simulink model "Mixture"  (Simulink 6.3)
settings: Solver=ode23s  StartTime=0  StopTime=800  MaxStep=0.1  RelTol=1e-3
undefined symbols (not defined in the file or in its folder): sigbuilder_block
Description:
  | This is a model of depression in synapses
settings Model: Creator=chchlee  LastModifiedBy=Owner  ExtModeAutoUpdateStatusClock=off
settings DataIOCC: SignalLoggingName=sigsOut
settings OptimizationCC: InlineInvariantSignals=on
settings DebuggingCC: SolverPrmCheckMsg=none
settings HardwareCC: TargetUnknown=on
settings GRTTargetCC: ModelReferenceCompliant=off  MatFileLogging=off

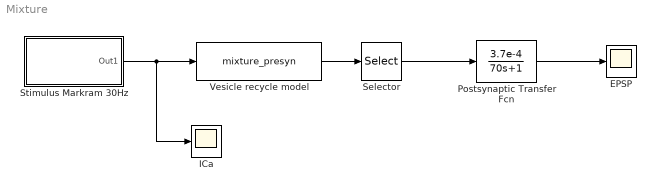
== system Mixture ==
  EPSP : Scope
      settings: TimeRange=600  YMin=-90  YMax=-76  SaveName=sim_mixture  DataFormat=Array
  ICa : Scope
      settings: YMin=-67.5  YMax=-63  SaveName=ScopeData3
  Postsynaptic Transfer Fcn : TransferFcn  Numerator=[3.7e-4]  Denominator=[70 1]
  Selector : Selector  Elements=[4]  InputPortWidth=4
  Stimulus Markram 30Hz : Subsystem
  Vesicle recycle model : S-Function  FunctionName=mixture_presyn
  wires:
  Selector/1 -> Postsynaptic Transfer Fcn/1
  Stimulus Markram 30Hz/1(Out1) -> ICa/1, Vesicle recycle model/1
  Vesicle recycle model/1 -> Selector/1
  Postsynaptic Transfer Fcn/1 -> EPSP/1

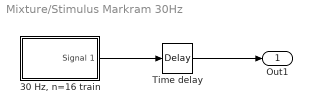
== system Mixture/Stimulus Markram 30Hz ==
  "30 Hz, n=16 train" : Subsystem  Tag=STV Subsys  LoadFcn=sigbuilder_block('load');  StartFcn=sigbuilder_block('start');  StopFcn=sigbuilder_block('stop');  ClipboardFcn=sigbuilder_block('clipboard');  mask(Sigbuilder block){}
      mask help: Sigbuilder GUI
      mask init:
      | if ~strcmp(get_param(bdroot(gcbh),'SimulationStatus'),'stopped') tuvar = sigbuilder_block('maskInit'); end
      settings: CopyFcn=sigbuilder_block('copy');  DeleteFcn=sigbuilder_block('delete');  ModelCloseFcn=sigbuilder_block('modelClose');  PreSaveFcn=sigbuilder_block('preSave');  NameChangeFcn=sigbuilder_block('namechange');  OpenFcn=sigbuilder_block('open',[-3 25.5 768 498 ]);  CloseFcn=sigbuilder_block('close');
      mask Display: plot(0,0,100,100,[10,10,40,40,10],[80,20,20,80,80],[40,10],[50,50], [40,27,10],[65,72,56],[40,25,25,10],[28,28,43,43]);
  Time delay : TransportDelay  DelayTime=60  BufferSize=2000
  Out1 : Outport
  wires:
  "30 Hz, n=16 train"/1(Signal 1) -> Time delay/1
  Time delay/1 -> Out1/1

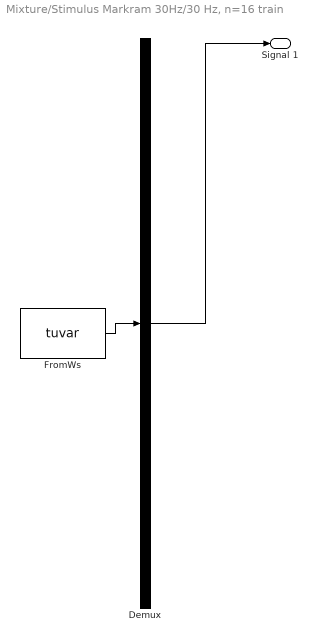
== system Mixture/Stimulus Markram 30Hz/30 Hz, n=16 train ==
  Demux : Demux  Tag=STV Demux  Outputs=1
  FromWs : FromWorkspace  Tag=STV FromWs  VariableName=tuvar  SampleTime=0  SigBuilderData=DataTag0  VnvData=DataTag1
      SigBuilderData=|
      | channels.label = 'Signal 1'
      | channels.allXData = {[0 0 1 1 33.3333333333 33.3333333333 34.3333333333 34.3333333333 66.6666666667 66.6666666667 67.6666666667 67.6666666667 100 100 101 101 133.333333333 133.333333333 134.333333333 134.333333333 166.666666667 166.666666667 167.666666667 167.666666667 200 200 201 201 233.333333333 233.333333333 234.333333333 234.333333333 266.666666667 266.666666667 267.666666667 267.666666667 300 300 301 301 333.333333333 333.333333333 334.333333333 334.333333333 366.666666667 366.666666667 367.666666667 367.666666667 400 400 401 401 433.333333333 433.333333333 434.333333333 434.333333333 466.666666667 466.666666667 467.666666667 467.666666667 500 500 501 501 533.333333333 533.333333333 534.333333333 540 640]}
      | channels.allYData = {[0 1 1 0 0 1 1 0 0 1 1 0 0 1 1 0 0 1 1 0 0 1 1 0 0 1 1 0 0 1 1 0 0 1 1 0 0 1 1 0 0 1 1 0 0 1 1 0 0 1 1 0 0 1 1 0 0 1 1 0 0 1 1 0 0 0 0 0 0]}
      | dataSet.timeRange = [0 640]
      | dataSet.name = 'Group 1'
  Signal 1 : Outport  Tag=STV Outport
  wires:
  Demux/1 -> Signal 1/1
  FromWs/1 -> Demux/1
